simulink model "Simulation"  (R2020a)
settings: Solver=VariableStepAuto  StartTime=0.0  StopTime=2  FixedStep=3e-5  RelTol=1e-3
values from neighbouring files (symbols this model uses):
  denom = Hs.Denominator{:}    [butterworthFilter.m]
  fs = omega_s * fp    [butterworthFilter.m]    (also in main.m = 10000; trem_por_sinal.m = 2000)
  Md = ceil(fs/(3 * (1000)))    [main.m]
  Mu = 1    [main.m]
  num = Hs.Numerator{:}    [butterworthFilter.m]
undefined symbols (not defined in the file or in its folder): designMultirateFIR
libraries: dspxfrm3 x9, dsparch4 x1, dspmlti4 x1
settings Model: Creator=victo  LastModifiedBy=victo
settings DataIOCC: ReturnWorkspaceOutputs=off

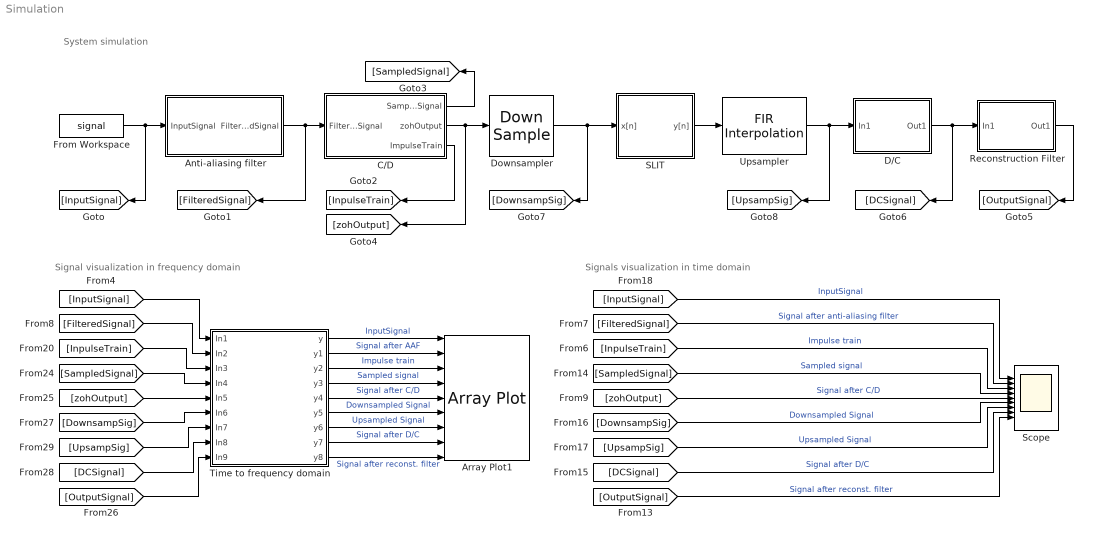
== system Simulation ==
  note: System simulation
  note: Signals visualization in time domain
  note: Signal visualization in frequency domain
  " C/D" : Subsystem
  Anti-aliasing filter : Subsystem
  Array Plot1 : ArrayPlot  NumInputPorts=9
  D/C : Subsystem
  Downsampler : DownSample  N=Md  RateOptions=Allow multirate processing
  From Workspace : FromWorkspace  VariableName=signal
  Reconstruction Filter : Subsystem
  SLIT : Subsystem
  Scope : Scope  NumInputPorts=9
  Time to frequency domain : Subsystem
  Upsampler : dspmlti4/FIR Interpolation  FilterSource=Auto  PrivateCoeffs=0  h=designMultirateFIR(3,1)  L=Mu  FilterObject=FINTERP  framing=Allow multirate processing  outputBufInitCond=0  roundingMode=Floor  overflowMode=off  firstCoeffDataTypeStr=Inherit: Same word length as input  firstCoeffMin=[]  firstCoeffMax=[]  firstCoeffLastDataTypeStr=Inherit: Same word length as input  outputDataTypeStr=Inherit: Same as accumulator  outputMin=[]  outputMax=[]  outputLastDataTypeStr=Inherit: Same as accumulator
  wires:
  Anti-aliasing filter/1(FilteredSignal) -> " C/D"/1(FilteredSignal), [FilteredSignal]
  " C/D"/3(ImpulseTrain) -> [InpulseTrain]
  " C/D"/1(SampledSignal) -> [SampledSignal]
  " C/D"/2(zohOutput) -> Downsampler/1, [zohOutput]
  From Workspace/1 -> Anti-aliasing filter/1(InputSignal), [InputSignal]
  SLIT/1(y[n]) -> Upsampler/1
  Upsampler/1 -> D/C/1(In1), [UpsampSig]
  D/C/1(Out1) -> Reconstruction Filter/1(In1), [DCSignal]
  Reconstruction Filter/1(Out1) -> [OutputSignal]
  [InpulseTrain] -> Scope/3  "Impulse train"
  [DownsampSig] -> Scope/6  "Downsampled Signal"
  [UpsampSig] -> Scope/7  "Upsampled Signal"
  [SampledSignal] -> Scope/4  "Sampled signal"
  [InputSignal] -> Scope/1  "InputSignal"
  [zohOutput] -> Scope/5  "Signal after C/D"
  [OutputSignal] -> Scope/9  "Signal after reconst. filter"
  [DCSignal] -> Scope/8  "Signal after D/C"
  [FilteredSignal] -> Scope/2  "Signal after anti-aliasing filter"
  Downsampler/1 -> SLIT/1(x[n]), [DownsampSig]
  [InputSignal] -> Time to frequency domain/1(In1)
  Time to frequency domain/1(y) -> Array Plot1/1  "InputSignal"
  Time to frequency domain/2(y1) -> Array Plot1/2  "Signal after AAF"
  Time to frequency domain/5(y4) -> Array Plot1/5  "Signal after C/D"
  Time to frequency domain/7(y6) -> Array Plot1/7  "Upsampled Signal"
  Time to frequency domain/8(y7) -> Array Plot1/8  "Signal after D/C"
  Time to frequency domain/6(y5) -> Array Plot1/6  "Downsampled Signal"
  Time to frequency domain/3(y2) -> Array Plot1/3  "Impulse train"
  Time to frequency domain/4(y3) -> Array Plot1/4  "Sampled signal"
  Time to frequency domain/9(y8) -> Array Plot1/9  "Signal after reconst. filter"
  [FilteredSignal] -> Time to frequency domain/2(In2)
  [InpulseTrain] -> Time to frequency domain/3(In3)
  [SampledSignal] -> Time to frequency domain/4(In4)
  [zohOutput] -> Time to frequency domain/5(In5)
  [DownsampSig] -> Time to frequency domain/6(In6)
  [UpsampSig] -> Time to frequency domain/7(In7)
  [DCSignal] -> Time to frequency domain/8(In8)
  [OutputSignal] -> Time to frequency domain/9(In9)

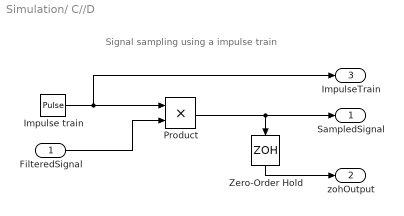
== system Simulation/ C//D ==
  note: Signal sampling using a impulse train
  FilteredSignal : Inport
  Impulse train : DiscretePulseGenerator  PulseType=Time based  Period=1/fs  PulseWidth=5
  Product : Product
  Zero-Order Hold : ZeroOrderHold  SampleTime=1/fs
  SampledSignal : Outport
  zohOutput : Outport  Port=2
  ImpulseTrain : Outport  Port=3
  wires:
  Impulse train/1 -> Product/1, ImpulseTrain/1
  Zero-Order Hold/1 -> zohOutput/1
  FilteredSignal/1 -> Product/2
  Product/1 -> Zero-Order Hold/1, SampledSignal/1

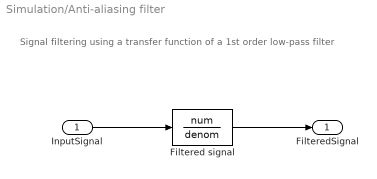
== system Simulation/Anti-aliasing filter ==
  note: Signal filtering using a transfer function of a 1st order low-pass filter
  InputSignal : Inport
  Filtered signal : TransferFcn  Numerator=num  Denominator=denom
  FilteredSignal : Outport
  wires:
  Filtered signal/1 -> FilteredSignal/1
  InputSignal/1 -> Filtered signal/1

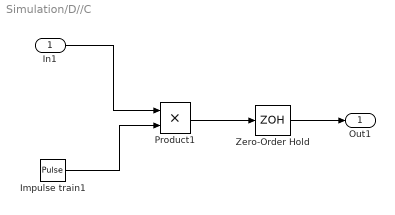
== system Simulation/D//C ==
  In1 : Inport
  Impulse train1 : DiscretePulseGenerator  PulseType=Time based  Period=1/((fs/Md)*Mu)  PulseWidth=5
  Product1 : Product
  Zero-Order Hold : ZeroOrderHold  SampleTime=1/((fs/Md)*Mu)
  Out1 : Outport
  wires:
  Impulse train1/1 -> Product1/2
  In1/1 -> Product1/1
  Zero-Order Hold/1 -> Out1/1
  Product1/1 -> Zero-Order Hold/1

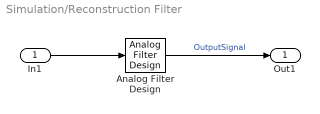
== system Simulation/Reconstruction Filter ==
  In1 : Inport
  Analog Filter Design : dsparch4/Analog Filter Design  method=Butterworth  filttype=Lowpass  N=8  Wlo=(fs/2)*2*pi  Whi=80  Rp=2  Rs=40
  Out1 : Outport
  wires:
  In1/1 -> Analog Filter Design/1
  Analog Filter Design/1 -> Out1/1  "OutputSignal"

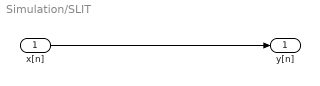
== system Simulation/SLIT ==
  x[n] : Inport
  y[n] : Outport
  wires:
  x[n]/1 -> y[n]/1

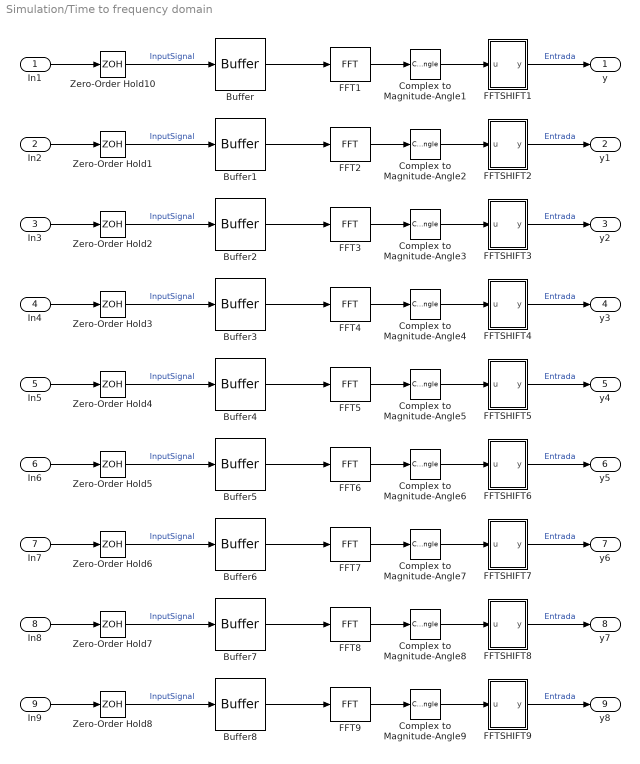
== system Simulation/Time to frequency domain ==
  In1 : Inport
  In2 : Inport  Port=2
  In3 : Inport  Port=3
  In4 : Inport  Port=4
  In5 : Inport  Port=5
  In6 : Inport  Port=6
  In7 : Inport  Port=7
  In8 : Inport  Port=8
  In9 : Inport  Port=9
  Buffer{,1..8} (9 alike) : Buffer  N=8192  OutputFrames=off
  Complex to Magnitude-Angle{1..9} (9 alike) : ComplexToMagnitudeAngle  Output=Magnitude
  FFT{1..9} (9 alike) : dspxfrm3/FFT  FFTImplementation=Auto  CompMethod=Table lookup  TableOpt=NEW  TableOptActive=Speed  BitRevOrder=off  Normalize=off  InheritFFTLength=on  FFTLength=64  WrapInput=on  roundingMode=Floor  overflowMode=off  firstCoeffDataTypeStr=Inherit: Same word length as input  firstCoeffLastDataTypeStr=Inherit: Same word length as input  outputMin=[]  outputMax=[]
  FFTSHIFT1 : MATLAB Function  TreatAsAtomicUnit=on
  FFTSHIFT2 : MATLAB Function  TreatAsAtomicUnit=on
  FFTSHIFT3 : MATLAB Function  TreatAsAtomicUnit=on
  FFTSHIFT4 : MATLAB Function  TreatAsAtomicUnit=on
  FFTSHIFT5 : MATLAB Function  TreatAsAtomicUnit=on
  FFTSHIFT6 : MATLAB Function  TreatAsAtomicUnit=on
  FFTSHIFT7 : MATLAB Function  TreatAsAtomicUnit=on
  FFTSHIFT8 : MATLAB Function  TreatAsAtomicUnit=on
  FFTSHIFT9 : MATLAB Function  TreatAsAtomicUnit=on
  Zero-Order Hold{1..8,10} (9 alike) : ZeroOrderHold  SampleTime=1/(4*fs)
  y : Outport
  y1 : Outport  Port=2
  y2 : Outport  Port=3
  y3 : Outport  Port=4
  y4 : Outport  Port=5
  y5 : Outport  Port=6
  y6 : Outport  Port=7
  y7 : Outport  Port=8
  y8 : Outport  Port=9
  wires:
  In1/1 -> Zero-Order Hold10/1
  Buffer/1 -> FFT1/1
  Complex to Magnitude-Angle1/1 -> FFTSHIFT1/1(u)
  FFT1/1 -> Complex to Magnitude-Angle1/1
  FFTSHIFT1/1(y) -> y/1  "Entrada"
  Zero-Order Hold10/1 -> Buffer/1  "InputSignal"
  Zero-Order Hold1/1 -> Buffer1/1  "InputSignal"
  In2/1 -> Zero-Order Hold1/1
  FFTSHIFT2/1(y) -> y1/1  "Entrada"
  Complex to Magnitude-Angle2/1 -> FFTSHIFT2/1(u)
  Buffer1/1 -> FFT2/1
  FFT2/1 -> Complex to Magnitude-Angle2/1
  Zero-Order Hold2/1 -> Buffer2/1  "InputSignal"
  In3/1 -> Zero-Order Hold2/1
  FFTSHIFT3/1(y) -> y2/1  "Entrada"
  Complex to Magnitude-Angle3/1 -> FFTSHIFT3/1(u)
  Buffer2/1 -> FFT3/1
  FFT3/1 -> Complex to Magnitude-Angle3/1
  Zero-Order Hold3/1 -> Buffer3/1  "InputSignal"
  In4/1 -> Zero-Order Hold3/1
  FFTSHIFT4/1(y) -> y3/1  "Entrada"
  Complex to Magnitude-Angle4/1 -> FFTSHIFT4/1(u)
  Buffer3/1 -> FFT4/1
  FFT4/1 -> Complex to Magnitude-Angle4/1
  Zero-Order Hold4/1 -> Buffer4/1  "InputSignal"
  In5/1 -> Zero-Order Hold4/1
  FFTSHIFT5/1(y) -> y4/1  "Entrada"
  Complex to Magnitude-Angle5/1 -> FFTSHIFT5/1(u)
  Buffer4/1 -> FFT5/1
  FFT5/1 -> Complex to Magnitude-Angle5/1
  Zero-Order Hold5/1 -> Buffer5/1  "InputSignal"
  In6/1 -> Zero-Order Hold5/1
  FFTSHIFT6/1(y) -> y5/1  "Entrada"
  Complex to Magnitude-Angle6/1 -> FFTSHIFT6/1(u)
  Buffer5/1 -> FFT6/1
  FFT6/1 -> Complex to Magnitude-Angle6/1
  Zero-Order Hold6/1 -> Buffer6/1  "InputSignal"
  In7/1 -> Zero-Order Hold6/1
  FFTSHIFT7/1(y) -> y6/1  "Entrada"
  Complex to Magnitude-Angle7/1 -> FFTSHIFT7/1(u)
  Buffer6/1 -> FFT7/1
  FFT7/1 -> Complex to Magnitude-Angle7/1
  Zero-Order Hold7/1 -> Buffer7/1  "InputSignal"
  In8/1 -> Zero-Order Hold7/1
  FFTSHIFT8/1(y) -> y7/1  "Entrada"
  Complex to Magnitude-Angle8/1 -> FFTSHIFT8/1(u)
  Buffer7/1 -> FFT8/1
  FFT8/1 -> Complex to Magnitude-Angle8/1
  Zero-Order Hold8/1 -> Buffer8/1  "InputSignal"
  In9/1 -> Zero-Order Hold8/1
  FFTSHIFT9/1(y) -> y8/1  "Entrada"
  Complex to Magnitude-Angle9/1 -> FFTSHIFT9/1(u)
  Buffer8/1 -> FFT9/1
  FFT9/1 -> Complex to Magnitude-Angle9/1

== matlab function Simulation/Time to frequency domain/FFTSHIFT2 ==
  data: u input; y output
function y = fcn(u)

y = fftshift(u);

== matlab function Simulation/Time to frequency domain/FFTSHIFT3 ==
  data: u input; y output
function y = fcn(u)

y = fftshift(u);

== matlab function Simulation/Time to frequency domain/FFTSHIFT4 ==
  data: u input; y output
function y = fcn(u)

y = fftshift(u);

== matlab function Simulation/Time to frequency domain/FFTSHIFT5 ==
  data: u input; y output
function y = fcn(u)

y = fftshift(u);

== matlab function Simulation/Time to frequency domain/FFTSHIFT6 ==
  data: u input; y output
function y = fcn(u)

y = fftshift(u);

== matlab function Simulation/Time to frequency domain/FFTSHIFT7 ==
  data: u input; y output
function y = fcn(u)

y = fftshift(u);

== matlab function Simulation/Time to frequency domain/FFTSHIFT8 ==
  data: u input; y output
function y = fcn(u)

y = fftshift(u);

== matlab function Simulation/Time to frequency domain/FFTSHIFT9 ==
  data: u input; y output
function y = fcn(u)

y = fftshift(u);

== matlab function Simulation/Time to frequency domain/FFTSHIFT1 ==
  data: u input; y output
function y = fcn(u)

y = fftshift(u);
